simulink model "dataTypeDiff"  (R2020b)
settings: Solver=VariableStepAuto  StartTime=0.0  StopTime=endTime  RelTol=1e-3
values from neighbouring files (symbols this model uses):
  simDataMax = inDataMax(n)    [dataTypeDiff_18bitFix_tb.m]    (also in dataTypeDiff_tb.m)
  simDataMin = inDataMin(n)    [dataTypeDiff_18bitFix_tb.m]    (also in dataTypeDiff_tb.m)
settings Model: Creator=amatsumo  LastModifiedBy=amatsumo
settings OptimizationCC: BlockReduction=off  ConditionallyExecuteInputs=off  DefaultParameterBehavior=Inlined
settings DebuggingCC: AlgebraicLoopMsg=error  SingleTaskRateTransMsg=error
settings HardwareCC: ProdBitPerPointer=32  ProdBitPerSizeT=32  ProdBitPerPtrDiffT=32  ProdLargestAtomicFloat=None  ProdIntDivRoundTo=Undefined  ProdEndianess=Unspecified  ProdWordSize=32  ProdHWDeviceType=ASIC/FPGA->ASIC/FPGA  TargetBitPerPointer=64  TargetBitPerSizeT=64  TargetBitPerPtrDiffT=64  TargetLongLongMode=on  TargetIntDivRoundTo=Zero  TargetEndianess=LittleEndian  TargetWordSize=64  TargetHWDeviceType=Custom Processor->MATLAB Host Computer  ProdEqTarget=off

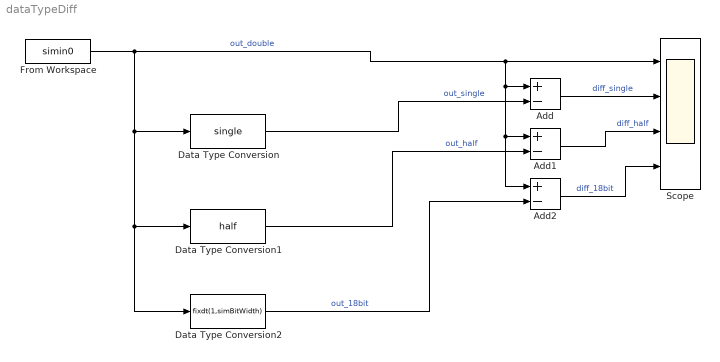
== system dataTypeDiff ==
  Add : Sum  Inputs=+-
  Add1 : Sum  Inputs=+-
  Add2 : Sum  Inputs=+-
  Data Type Conversion : DataTypeConversion  OutDataTypeStr=single  RndMeth=Convergent
  Data Type Conversion1 : DataTypeConversion  OutDataTypeStr=half  RndMeth=Convergent
  Data Type Conversion2 : DataTypeConversion  OutMin=simDataMin  OutMax=simDataMax  OutDataTypeStr=fixdt(1,simBitWidth)  RndMeth=Convergent
  From Workspace : FromWorkspace  VariableName=simin0  SampleTime=1
  Scope : Scope  NumInputPorts=4
  wires:
  From Workspace/1 -> Add2/1, Add1/1, Add/1, Scope/1, Data Type Conversion2/1, Data Type Conversion1/1, Data Type Conversion/1  "out_double"
  Add/1 -> Scope/2  "diff_single"
  Add1/1 -> Scope/3  "diff_half"
  Add2/1 -> Scope/4  "diff_18bit"
  Data Type Conversion/1 -> Add/2  "out_single"
  Data Type Conversion1/1 -> Add1/2  "out_half"
  Data Type Conversion2/1 -> Add2/2  "out_18bit"
